simulink model "act1_simulink_sesion3"  (R2020a)
settings: Solver=ode1  StartTime=0.0  StopTime=3  FixedStep=0.001  RelTol=1e-3
libraries: simulink_need_slupdate x6
settings Model: Creator=jaguero  LastModifiedBy=spide

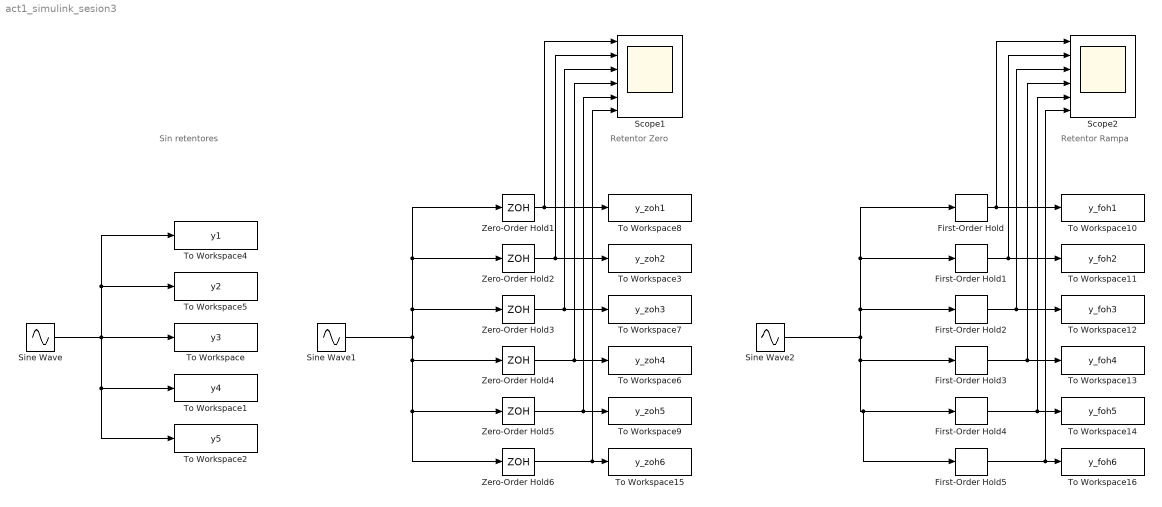
== system act1_simulink_sesion3 ==
  note: Sin retentores
  note: Retentor Zero
  note: Retentor Rampa
  First-Order Hold : simulink_need_slupdate/First-Order Hold  DisableCoverage=on  Ts=0.75
      settings: SourceProductBaseCode=SL
  First-Order Hold1 : simulink_need_slupdate/First-Order Hold  DisableCoverage=on  Ts=0.5
      settings: SourceProductBaseCode=SL
  First-Order Hold2 : simulink_need_slupdate/First-Order Hold  DisableCoverage=on  Ts=0.2
      settings: SourceProductBaseCode=SL
  First-Order Hold3 : simulink_need_slupdate/First-Order Hold  DisableCoverage=on  Ts=0.1
      settings: SourceProductBaseCode=SL
  First-Order Hold4 : simulink_need_slupdate/First-Order Hold  DisableCoverage=on  Ts=0.05
      settings: SourceProductBaseCode=SL
  First-Order Hold5 : simulink_need_slupdate/First-Order Hold  DisableCoverage=on  Ts=0.01
      settings: SourceProductBaseCode=SL
  Scope1 : Scope  NumInputPorts=6
  Scope2 : Scope  NumInputPorts=6
  Sine Wave : Sin  Frequency=2*pi  SampleTime=0
  Sine Wave1 : Sin  Frequency=2*pi  SampleTime=0
  Sine Wave2 : Sin  Frequency=2*pi  SampleTime=0
  To Workspace : ToWorkspace  VariableName=y3  SaveFormat=Timeseries  SampleTime=0.5
  To Workspace1 : ToWorkspace  VariableName=y4  SaveFormat=Timeseries  SampleTime=0.49
  To Workspace10 : ToWorkspace  VariableName=y_foh1  SaveFormat=Timeseries  SampleTime=-1
  To Workspace11 : ToWorkspace  VariableName=y_foh2  SaveFormat=Timeseries  SampleTime=-1
  To Workspace12 : ToWorkspace  VariableName=y_foh3  SaveFormat=Timeseries  SampleTime=-1
  To Workspace13 : ToWorkspace  VariableName=y_foh4  SaveFormat=Timeseries  SampleTime=-1
  To Workspace14 : ToWorkspace  VariableName=y_foh5  SaveFormat=Timeseries  SampleTime=-1
  To Workspace15 : ToWorkspace  VariableName=y_zoh6  SaveFormat=Timeseries  SampleTime=0.001
  To Workspace16 : ToWorkspace  VariableName=y_foh6  SaveFormat=Timeseries  SampleTime=-1
  To Workspace2 : ToWorkspace  VariableName=y5  SaveFormat=Timeseries  SampleTime=0.1
  To Workspace3 : ToWorkspace  VariableName=y_zoh2  SaveFormat=Timeseries  SampleTime=0.001
  To Workspace4 : ToWorkspace  VariableName=y1  SaveFormat=Timeseries  SampleTime=-1
  To Workspace5 : ToWorkspace  VariableName=y2  SaveFormat=Timeseries  SampleTime=0.51
  To Workspace6 : ToWorkspace  VariableName=y_zoh4  SaveFormat=Timeseries  SampleTime=0.001
  To Workspace7 : ToWorkspace  VariableName=y_zoh3  SaveFormat=Timeseries  SampleTime=0.001
  To Workspace8 : ToWorkspace  VariableName=y_zoh1  SaveFormat=Timeseries  SampleTime=0.001
  To Workspace9 : ToWorkspace  VariableName=y_zoh5  SaveFormat=Timeseries  SampleTime=0.001
  Zero-Order Hold1 : ZeroOrderHold  SampleTime=0.75
  Zero-Order Hold2 : ZeroOrderHold  SampleTime=0.5
  Zero-Order Hold3 : ZeroOrderHold  SampleTime=0.2
  Zero-Order Hold4 : ZeroOrderHold  SampleTime=0.1
  Zero-Order Hold5 : ZeroOrderHold  SampleTime=0.05
  Zero-Order Hold6 : ZeroOrderHold  SampleTime=0.01
  wires:
  Sine Wave1/1 -> Zero-Order Hold3/1, Zero-Order Hold2/1, Zero-Order Hold1/1, Zero-Order Hold6/1, Zero-Order Hold5/1, Zero-Order Hold4/1
  First-Order Hold1/1 -> Scope2/2, To Workspace11/1
  First-Order Hold2/1 -> Scope2/3, To Workspace12/1
  First-Order Hold3/1 -> Scope2/4, To Workspace13/1
  Sine Wave2/1 -> First-Order Hold2/1, First-Order Hold1/1, First-Order Hold/1, First-Order Hold5/1, First-Order Hold4/1, First-Order Hold3/1
  First-Order Hold4/1 -> Scope2/5, To Workspace14/1
  First-Order Hold5/1 -> Scope2/6, To Workspace16/1
  First-Order Hold/1 -> Scope2/1, To Workspace10/1
  Zero-Order Hold1/1 -> Scope1/1, To Workspace8/1
  Zero-Order Hold6/1 -> Scope1/6, To Workspace15/1
  Zero-Order Hold5/1 -> Scope1/5, To Workspace9/1
  Zero-Order Hold4/1 -> Scope1/4, To Workspace6/1
  Zero-Order Hold3/1 -> Scope1/3, To Workspace7/1
  Zero-Order Hold2/1 -> Scope1/2, To Workspace3/1
  Sine Wave/1 -> To Workspace4/1, To Workspace5/1, To Workspace/1, To Workspace2/1, To Workspace1/1
